simulink model "drone_failure_v3"  (R2021a)
settings: Solver=ode15s  StartTime=0.0  StopTime=35  FixedStep=0.1  RelTol=1e-3  EnableMultiTasking=on
settings Model: EnablePacing=on  PacingRate=1.100000  Creator=glembrez  LastModifiedBy=gabin
settings SolverCC: ZeroCrossAlgorithm=Adaptive  AlgebraicLoopSolver=TrustRegion  AutoInsertRateTranBlk=on
settings DataIOCC: LimitDataPoints=on
settings OptimizationCC: LifeSpan=inf
settings DebuggingCC: AllowSymbolicDim=off  SFUnexpectedBacktrackingDiag=warning  SFNoUnconditionalDefaultTransitionDiag=warning  SFExecutionAtInitializationDiag=none  ArithmeticOperatorsInVariantConditions=warning
settings SFSimCC: SimUseLocalCustomCode=off  CustomCodeUndefinedFunction=UseInterfaceOnly
settings RTWCC: RTWUseLocalCustomCode=off
settings CodeAppCC: StateflowObjectComments=on
settings GRTTargetCC: TargetLangStandard=C89/C90 (ANSI)
settings ConfigComp: CovMetricSettings=dw  CovSaveCumulativeToWorkspaceVar=on  CovSaveSingleToWorkspaceVar=on  CovExternalEMLEnable=off  CovSFcnEnable=off

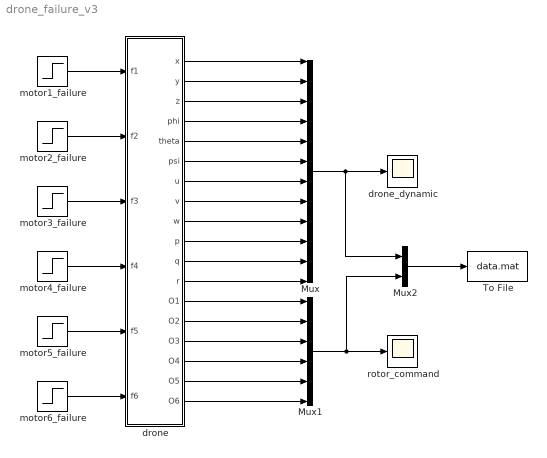
== system drone_failure_v3 ==
  Mux : Mux  Inputs=12
  Mux1 : Mux  Inputs=6
  Mux2 : Mux  Inputs=2
  To File : ToFile  Filename=data.mat  MatrixName=X  SaveFormat=Timeseries
  drone : Stateflow chart  TreatAsAtomicUnit=on
  drone_dynamic : Scope
  motor1_failure : Step  Time=10  SampleTime=0
  motor2_failure : Step  Time=35  SampleTime=0
  motor3_failure : Step  Time=35  SampleTime=0
  motor4_failure : Step  Time=35  SampleTime=0
  motor5_failure : Step  Time=35  SampleTime=0
  motor6_failure : Step  Time=35  SampleTime=0
  rotor_command : Scope
  wires:
  drone/1(x) -> Mux/1
  Mux/1 -> Mux2/1, drone_dynamic/1
  drone/2(y) -> Mux/2
  drone/3(z) -> Mux/3
  drone/4(phi) -> Mux/4
  drone/5(theta) -> Mux/5
  drone/6(psi) -> Mux/6
  drone/7(u) -> Mux/7
  drone/8(v) -> Mux/8
  drone/9(w) -> Mux/9
  drone/10(p) -> Mux/10
  drone/11(q) -> Mux/11
  drone/12(r) -> Mux/12
  drone/13(O1) -> Mux1/1
  drone/14(O2) -> Mux1/2
  drone/15(O3) -> Mux1/3
  drone/16(O4) -> Mux1/4
  drone/17(O5) -> Mux1/5
  drone/18(O6) -> Mux1/6
  Mux1/1 -> Mux2/2, rotor_command/1
  Mux2/1 -> To File/1
  motor2_failure/1 -> drone/2(f2)
  motor3_failure/1 -> drone/3(f3)
  motor4_failure/1 -> drone/4(f4)
  motor5_failure/1 -> drone/5(f5)
  motor6_failure/1 -> drone/6(f6)
  motor1_failure/1 -> drone/1(f1)

== stateflow chart drone_failure_v3/drone ==
  settings: updateMethod=CONTINUOUS
  state Drone
    state Normal_flight [parallel]
      %drone dynamic
      during:
      x_dot = cos(theta)*cos(psi)*u + (cos(psi)*sin(phi)*sin(theta)-cos(psi)*cos(phi))*v + (sin(phi)*sin(psi)+cos(phi)*cos(psi)*sin(theta))*w ;
      y_dot = cos(theta)*sin(psi)*u + (cos(theta)*cos(psi)+sin(phi)*sin(theta)*sin(psi))*v + (cos(phi)*sin(theta)*sin(psi)-sin(phi)*cos(psi))*w ;
      z_dot = -sin(theta)*u + cos(theta)*sin(phi)*v + cos(theta)*cos(phi)*w ;
      phi_dot = p+sin(phi)*tan(theta)*q+cos(phi)*tan(theta)*r ;
      theta_dot = cos(phi)*q - sin(phi)*r ;
      psi_dot = q*sin(phi)/cos(theta) + r*cos(phi)/cos(theta) ;
      u_dot = v*r-q*w-g*sin(theta)-u*(Kt+Kd*sqrt(u^2+v^2+w^2))/m ;
      v_dot = p*w-r*u+g*sin(phi)*cos(theta)-v*(Kt+Kd*sqrt(u^2+v^2+w^2))/m ;
      w_dot =q*u-p*v+g*cos(phi)*cos(theta)-w*Kd*sqrt(u^2+v^2+w^2)/m-(b*(O1^4+O2^4+O3^4+O4^4+O5^4+O6^4))/m;
      p_dot = q*r*(Iyy-Izz)/Ixx +((b*l/2 * (2*O2^4-2*O5^4+O1^4+O3^4-O4^4-O6^4))...
      -Jr*q*(-O1^2+O2^2-O3^2+O4^2-O5^2+O6^2))/Ixx;
      q_dot = p*r*(Izz-Ixx)/Iyy+((sqrt(3)*b*l/2 * (O1^4+O6^4-O3^4-O4^4))...
      +Jr*p*(-O1^2+O2^2-O3^2+O4^2-O5^2+O6^2))/Iyy ;
      r_dot = p*q*(Ixx-Iyy)/Izz+ (d*(O1^4-O2^4+O3^4-O4^4+O5^4-O6^4)...
      -Jr*2*(-O1*(O1c - O1)/0.01+O2*(O2c - O2)/0.01-O3*(O3c - O3)/0.01...
      +O4*(O4c - O4)/0.01-O5*(O5c - O5)/0.01+O6*(O6c - O6)/0.01))/Izz ;
      settings: executionOrder=1
    state Failure_detection [parallel]
      settings: executionOrder=2
      state fail4and2
        during:
        O1_dot = (O1c - O1)/tau+Kz*z-Kphi*phi+Ktheta*theta ;
        O2_dot = (O2c - O2)/tau ;
        O3_dot = (O3c - O3)/tau+Kz*z-Kphi*phi-Ktheta*theta ;
        O4_dot = (O4c - O4)/tau ;
        O5_dot = (O5c - O5)/tau +Kz*z+Kphi*phi ;;
        O6_dot = (O6c - O6)/tau+Kz*z+Kphi*phi+Ktheta*theta ;
      state fail1and5
        during:
        O1_dot = (O1c - O1)/tau ;
        O2_dot = (O2c - O2)/tau+Kz*z-Kphi*phi ;
        O3_dot = (O3c - O3)/tau+Kz*z-Kphi*phi-Ktheta*theta ;
        O4_dot = (O4c - O4)/tau+Kz*z-Kphi*phi-Ktheta*theta ;
        O5_dot = (O5c - O5)/tau ;
        O6_dot = (O6c - O6)/tau+Kz*z+Kphi*phi+Ktheta*theta ;
      state fail4
        during:
        O1_dot = (O1c - O1)/tau ;
        O2_dot = (O2c - O2)/tau+Kz*z-Kphi*phi ;
        O3_dot = (O3c - O3)/tau+Kz*z-Kphi*phi-Ktheta*theta ;
        O4_dot = (O4c - O4)/tau ;
        O5_dot = (O5c - O5)/tau+Kz*z+Kphi*phi ;
        O6_dot = (O6c - O6)/tau+Kz*z+Kphi*phi+Ktheta*theta ;
      state fail1
        during:
        O1_dot = (O1c - O1)/tau ;
        O2_dot = (O2c - O2)/tau+Kz*z-Kphi*phi ;
        O3_dot = (O3c - O3)/tau+Kz*z-Kphi*phi-Ktheta*theta ;
        O4_dot = (O4c - O4)/tau ;
        O5_dot = (O5c - O5)/tau+Kz*z+Kphi*phi ;
        O6_dot = (O6c - O6)/tau+Kz*z+Kphi*phi+Ktheta*theta ;
      state fail4and6
        during:
        O1_dot = (O1c - O1)/tau+Kz*z-Kphi*phi+Ktheta*theta ;
        O2_dot = (O2c - O2)/tau ;
        O3_dot = (O3c - O3)/tau+Kz*z-Kphi*phi-Ktheta*theta ;
        O4_dot = (O4c - O4)/tau ;
        O5_dot = (O5c - O5)/tau +Kz*z+Kphi*phi ;;
        O6_dot = (O6c - O6)/tau+Kz*z+Kphi*phi+Ktheta*theta ;
      state fail1and3
        during:
        O1_dot = (O1c - O1)/tau ;
        O2_dot = (O2c - O2)/tau+Kz*z-Kphi*phi ;
        O3_dot = (O3c - O3)/tau  ;
        O4_dot = (O4c - O4)/tau+Kz*z-Kphi*phi-Ktheta*theta ;
        O5_dot = (O5c - O5)/tau+Kz*z+Kphi*phi ;
        O6_dot = (O6c - O6)/tau+Kz*z+Kphi*phi+Ktheta*theta ;
      state fail2and4
        during:
        O1_dot = (O1c - O1)/tau+Kz*z-Kphi*phi+Ktheta*theta ;
        O2_dot = (O2c - O2)/tau ;
        O3_dot = (O3c - O3)/tau+Kz*z-Kphi*phi-Ktheta*theta ;
        O4_dot = (O4c - O4)/tau ;
        O5_dot = (O5c - O5)/tau +Kz*z+Kphi*phi ;;
        O6_dot = (O6c - O6)/tau+Kz*z+Kphi*phi+Ktheta*theta ;
      state fail5and1
        during:
        O1_dot = (O1c - O1)/tau ;
        O2_dot = (O2c - O2)/tau+Kz*z-Kphi*phi ;
        O3_dot = (O3c - O3)/tau+Kz*z-Kphi*phi-Ktheta*theta ;
        O4_dot = (O4c - O4)/tau+Kz*z-Kphi*phi-Ktheta*theta ;
        O5_dot = (O5c - O5)/tau ;
        O6_dot = (O6c - O6)/tau+Kz*z+Kphi*phi+Ktheta*theta ;
      state P_correction
        during:
        O1_dot = (O1c - O1)/tau+Kz*z-Kphi*phi+Ktheta*theta ;
        O2_dot = (O2c - O2)/tau+Kz*z-Kphi*phi ;
        O3_dot = (O3c - O3)/tau+Kz*z-Kphi*phi-Ktheta*theta ;
        O4_dot = (O4c - O4)/tau+Kz*z+Kphi*phi-Ktheta*theta ;
        O5_dot = (O5c - O5)/tau+Kz*z+Kphi*phi ;
        O6_dot = (O6c - O6)/tau+Kz*z+Kphi*phi+Ktheta*theta;
      state fail5
        during:
        O1_dot = (O1c - O1)/tau+Kz*z-Kphi*phi+Ktheta*theta ;
        O2_dot = (O2c - O2)/tau ;
        O3_dot = (O3c - O3)/tau+Kz*z-Kphi*phi-Ktheta*theta ;
        O4_dot = (O4c - O4)/tau+Kz*z+Kphi*phi-Ktheta*theta ;
        O5_dot = (O5c - O5)/tau ;
        O6_dot = (O6c - O6)/tau+Kz*z+Kphi*phi+Ktheta*theta ;
      state uncontrolable1
        during:
        O1_dot = (O1c - O1)/tau ;
        O2_dot = (O2c - O2)/tau ;
        O3_dot = (O3c - O3)/tau ;
        O4_dot = (O4c - O4)/tau ;
        O5_dot = (O5c - O5)/tau ;
        O6_dot = (O6c - O6)/tau;
      state fail2
        during:
        O1_dot = (O1c - O1)/tau+Kz*z-Kphi*phi+Ktheta*theta ;
        O2_dot = (O2c - O2)/tau ;
        O3_dot = (O3c - O3)/tau+Kz*z-Kphi*phi-Ktheta*theta ;
        O4_dot = (O4c - O4)/tau+Kz*z+Kphi*phi-Ktheta*theta ;
        O5_dot = (O5c - O5)/tau ;
        O6_dot = (O6c - O6)/tau+Kz*z+Kphi*phi+Ktheta*theta ;
      state uncontrolable
        during:
        O1_dot = (O1c - O1)/tau ;
        O2_dot = (O2c - O2)/tau ;
        O3_dot = (O3c - O3)/tau ;
        O4_dot = (O4c - O4)/tau ;
        O5_dot = (O5c - O5)/tau ;
        O6_dot = (O6c - O6)/tau;
      state fail5and3
        during:
        O1_dot = (O1c - O1)/tau+Kz*z-Kphi*phi+Ktheta*theta ;
        O2_dot = (O2c - O2)/tau+Kz*z-Kphi*phi ;
        O3_dot = (O3c - O3)/tau ;
        O4_dot = (O4c - O4)/tau+Kz*z+Kphi*phi-Ktheta*theta ;
        O5_dot = (O5c - O5)/tau ;
        O6_dot = (O6c - O6)/tau+Kz*z+Kphi*phi+Ktheta*theta ;
      state fail2and6
        during:
        O1_dot = (O1c - O1)/tau+Kz*z-Kphi*phi+Ktheta*theta ;
        O2_dot = (O2c - O2)/tau ;
        O3_dot = (O3c - O3)/tau+Kz*z-Kphi*phi-Ktheta*theta ;
        O4_dot = (O4c - O4)/tau+Kz*z+Kphi*phi-Ktheta*theta ;
        O5_dot = (O5c - O5)/tau +Kz*z+Kphi*phi ;
        O6_dot = (O6c - O6)/tau ;
      state fail3and1
        during:
        O1_dot = (O1c - O1)/tau ;
        O2_dot = (O2c - O2)/tau+Kz*z-Kphi*phi ;
        O3_dot = (O3c - O3)/tau  ;
        O4_dot = (O4c - O4)/tau+Kz*z-Kphi*phi-Ktheta*theta ;
        O5_dot = (O5c - O5)/tau+Kz*z+Kphi*phi ;
        O6_dot = (O6c - O6)/tau+Kz*z+Kphi*phi+Ktheta*theta ;
      state fail6and2
        during:
        O1_dot = (O1c - O1)/tau+Kz*z-Kphi*phi+Ktheta*theta ;
        O2_dot = (O2c - O2)/tau ;
        O3_dot = (O3c - O3)/tau+Kz*z-Kphi*phi-Ktheta*theta ;
        O4_dot = (O4c - O4)/tau+Kz*z+Kphi*phi-Ktheta*theta ;
        O5_dot = (O5c - O5)/tau +Kz*z+Kphi*phi ;
        O6_dot = (O6c - O6)/tau ;
      state fail6
        during:
        O1_dot = (O1c - O1)/tau+Kz*z-Kphi*phi+Ktheta*theta ;
        O2_dot = (O2c - O2)/tau+Kz*z-Kphi*phi ;
        O3_dot = (O3c - O3)/tau ;
        O4_dot = (O4c - O4)/tau+Kz*z+Kphi*phi-Ktheta*theta ;
        O5_dot = (O5c - O5)/tau+Kz*z+Kphi*phi ;
        O6_dot = (O6c - O6)/tau ;
      state fail3
        during:
        O1_dot = (O1c - O1)/tau+Kz*z-Kphi*phi+Ktheta*theta ;
        O2_dot = (O2c - O2)/tau+Kz*z-Kphi*phi ;
        O3_dot = (O3c - O3)/tau ;
        O4_dot = (O4c - O4)/tau+Kz*z+Kphi*phi-Ktheta*theta ;
        O5_dot = (O5c - O5)/tau+Kz*z+Kphi*phi ;
        O6_dot = (O6c - O6)/tau ;
      state fail3and5
        during:
        O1_dot = (O1c - O1)/tau+Kz*z-Kphi*phi+Ktheta*theta ;
        O2_dot = (O2c - O2)/tau+Kz*z-Kphi*phi ;
        O3_dot = (O3c - O3)/tau ;
        O4_dot = (O4c - O4)/tau+Kz*z+Kphi*phi-Ktheta*theta ;
        O5_dot = (O5c - O5)/tau ;
        O6_dot = (O6c - O6)/tau+Kz*z+Kphi*phi+Ktheta*theta ;
      state fail6and4
        during:
        O1_dot = (O1c - O1)/tau+Kz*z-Kphi*phi+Ktheta*theta ;
        O2_dot = (O2c - O2)/tau ;
        O3_dot = (O3c - O3)/tau+Kz*z-Kphi*phi-Ktheta*theta ;
        O4_dot = (O4c - O4)/tau ;
        O5_dot = (O5c - O5)/tau +Kz*z+Kphi*phi ;
        O6_dot = (O6c - O6)/tau+Kz*z+Kphi*phi+Ktheta*theta ;
      fail4and2 -> uncontrolable1 : [f1>eps|...
          | f6>eps|...
          | f3>eps|...
          | f5>eps]
          | {O1c= 0;
          | O2c = 0;
          | O3c = 0;
          | O4c = 0;
          | O5c = 0;
          | O6c = 0}
      fail1and5 -> uncontrolable : [f3>eps|...
          | f4>eps|...
          | f2>eps|...
          | f6>eps]
          | {O1c= 0;
          | O2c = 0;
          | O3c = 0;
          | O4c = 0;
          | O5c = 0;
          | O6c = 0}
      fail4 -> fail4and2 [order 1] : [f2>eps]{O1c=(m*g/(5*b))^(1/4);
          | O2c = 0;
          | O3c = (2^(1/4))*(m*g/(5*b))^(1/4);
          | O4c =  0;
          | O5c = (m*g/(5*b))^(1/4);
          | O6c = (m*g/(5*b))^(1/4)}
      fail1 -> fail1and5 [order 1] : [f5>eps]{O1c=0;
          | O2c = (m*g/(5*b))^(1/4);
          | O3c = (m*g/(5*b))^(1/4);
          | O4c =  (m*g/(5*b))^(1/4);
          | O5c = 0;
          | O6c = (2^(1/4))*(m*g/(5*b))^(1/4)}
      fail1 -> fail1 [order 4] : [f4>eps]
      fail4 -> uncontrolable1 [order 3] : [f3>eps|...
          | f5>eps]
          | {O1c= 0;
          | O2c = 0;
          | O3c = 0;
          | O4c = 0;
          | O5c = 0;
          | O6c = 0}
      P_correction -> fail1 [order 1] : [f1>eps]{O1c=0;
          | O2c = (m*g/(4*b))^(1/4);
          | O3c = (m*g/(4*b))^(1/4);
          | O4c = 0;
          | O5c = (m*g/(4*b))^(1/4);
          | O6c = (m*g/(4*b))^(1/4)}
      P_correction -> fail4 [order 4] : [f4>eps]{O1c=0;
          | O2c = (m*g/(4*b))^(1/4);
          | O3c = (m*g/(4*b))^(1/4);
          | O4c = 0;
          | O5c = (m*g/(4*b))^(1/4);
          | O6c = (m*g/(4*b))^(1/4)}
      fail1 -> uncontrolable [order 3] : [f6>eps|...
          | f2>eps]
          | {O1c= 0;
          | O2c = 0;
          | O3c = 0;
          | O4c = 0;
          | O5c = 0;
          | O6c = 0}
      fail4 -> fail4and6 [order 2] : [f6>eps]{O1c=(m*g/(5*b))^(1/4);
          | O2c = 0;
          | O3c = (m*g/(5*b))^(1/4);
          | O4c =  (m*g/(5*b))^(1/4);
          | O5c = (2^(1/4))*(m*g/(5*b))^(1/4);
          | O6c = 0}
      fail4 -> fail4 [order 4] : [f1>eps]
      fail1 -> fail1and3 [order 2] : [f3>eps]{O1c=0;
          | O2c = (2^(1/4))*(m*g/(5*b))^(1/4);
          | O3c = 0;
          | O4c =  (m*g/(5*b))^(1/4);
          | O5c = (m*g/(5*b))^(1/4);
          | O6c = (m*g/(5*b))^(1/4)}
      fail4and6 -> uncontrolable1 : [f1>eps|...
          | f2>eps|...
          | f3>eps|...
          | f5>eps]
          | {O1c= 0;
          | O2c = 0;
          | O3c = 0;
          | O4c = 0;
          | O5c = 0;
          | O6c = 0}
      fail1and3 -> uncontrolable : [f4>eps|...
          | f5>eps|...
          | f2>eps|...
          | f6>eps]
          | {O1c= 0;
          | O2c = 0;
          | O3c = 0;
          | O4c = 0;
          | O5c = 0;
          | O6c = 0}
      fail5 -> fail5and1 [order 1] : [f1>eps]{O1c=0;
          | O2c = (m*g/(5*b))^(1/4);
          | O3c = (m*g/(5*b))^(1/4);
          | O4c =  (m*g/(5*b))^(1/4);
          | O5c = 0;
          | O6c = (2^(1/4))*(m*g/(5*b))^(1/4)}
      fail2 -> fail2and4 [order 1] : [f4>eps]{O1c=(m*g/(5*b))^(1/4);
          | O2c = 0;
          | O3c = (2^(1/4))*(m*g/(5*b))^(1/4);
          | O4c =  0;
          | O5c = (m*g/(5*b))^(1/4);
          | O6c = (m*g/(5*b))^(1/4)}
      fail2 -> fail2 [order 4] : [f5>eps]
      fail5and1 -> uncontrolable1 : [f2>eps|...
          | f3>eps|...
          | f4>eps|...
          | f6>eps]
          | {O1c= 0;
          | O2c = 0;
          | O3c = 0;
          | O4c = 0;
          | O5c = 0;
          | O6c = 0}
      fail2and4 -> uncontrolable : [f5>eps|...
          | f6>eps|...
          | f1>eps|...
          | f3>eps]
          | {O1c= 0;
          | O2c = 0;
          | O3c = 0;
          | O4c = 0;
          | O5c = 0;
          | O6c = 0}
      (default) -> P_correction
      fail5 -> uncontrolable1 [order 3] : [f6>eps|...
          | f4>eps]
          | {O1c= 0;
          | O2c = 0;
          | O3c = 0;
          | O4c = 0;
          | O5c = 0;
          | O6c = 0}
      P_correction -> fail5 [order 5] : [f5>eps]{O1c=(m*g/(4*b))^(1/4);
          | O2c = 0;
          | O3c =  (m*g/(4*b))^(1/4);
          | O4c = (m*g/(4*b))^(1/4);
          | O5c = 0;
          | O6c = (m*g/(4*b))^(1/4)}
      fail5and3 -> uncontrolable1 : [f1>eps|...
          | f2>eps|...
          | f4>eps|...
          | f6>eps]
          | {O1c= 0;
          | O2c = 0;
          | O3c = 0;
          | O4c = 0;
          | O5c = 0;
          | O6c = 0}
      fail2 -> uncontrolable [order 3] : [f3>eps|...
          | f1>eps]
          | {O1c= 0;
          | O2c = 0;
          | O3c = 0;
          | O4c = 0;
          | O5c = 0;
          | O6c = 0}
      fail2and6 -> uncontrolable : [f4>eps|...
          | f5>eps|...
          | f1>eps|...
          | f3>eps]
          | {O1c= 0;
          | O2c = 0;
          | O3c = 0;
          | O4c = 0;
          | O5c = 0;
          | O6c = 0}
      P_correction -> fail2 [order 2] : [f2>eps]{O1c=(m*g/(4*b))^(1/4);
          | O2c = 0;
          | O3c =  (m*g/(4*b))^(1/4);
          | O4c = (m*g/(4*b))^(1/4);
          | O5c = 0;
          | O6c = (m*g/(4*b))^(1/4)}
      fail6 -> uncontrolable1 [order 3] : [f1>eps|...
          | f5>eps]
          | {O1c= 0;
          | O2c = 0;
          | O3c = 0;
          | O4c = 0;
          | O5c = 0;
          | O6c = 0}
      fail6and2 -> uncontrolable1 : [f1>eps|...
          | f3>eps|...
          | f4>eps|...
          | f5>eps]
          | {O1c= 0;
          | O2c = 0;
          | O3c = 0;
          | O4c = 0;
          | O5c = 0;
          | O6c = 0}
      fail6and4 -> uncontrolable1 : [f1>eps|...
          | f2>eps|...
          | f3>eps|...
          | f5>eps]
          | {O1c= 0;
          | O2c = 0;
          | O3c = 0;
          | O4c = 0;
          | O5c = 0;
          | O6c = 0}
      fail5 -> fail5and3 [order 2] : [f3>eps]{O1c=(m*g/(5*b))^(1/4);
          | O2c = (m*g/(5*b))^(1/4);
          | O3c = 0;
          | O4c = (2^(1/4))*(m*g/(5*b))^(1/4);
          | O5c = 0;
          | O6c = (m*g/(5*b))^(1/4)}
      fail5 -> fail5 [order 4] : [f2>eps]
      P_correction -> fail6 [order 6] : [f6>eps]{O1c=(m*g/(4*b))^(1/4);
          | O2c = (m*g/(4*b))^(1/4);
          | O3c = 0;
          | O4c = (m*g/(4*b))^(1/4);
          | O5c = (m*g/(4*b))^(1/4);
          | O6c = 0}
      P_correction -> fail3 [order 3] : [f3>eps]{O1c=(m*g/(4*b))^(1/4);
          | O2c = (m*g/(4*b))^(1/4);
          | O3c = 0;
          | O4c = (m*g/(4*b))^(1/4);
          | O5c = (m*g/(4*b))^(1/4);
          | O6c = 0}
      fail3 -> uncontrolable [order 4] : [f2>eps|...
          | f4>eps]
          | {O1c= 0;
          | O2c = 0;
          | O3c = 0;
          | O4c = 0;
          | O5c = 0;
          | O6c = 0}
      fail3and1 -> uncontrolable : [f5>eps|...
          | f6>eps|...
          | f2>eps|...
          | f4>eps]
          | {O1c= 0;
          | O2c = 0;
          | O3c = 0;
          | O4c = 0;
          | O5c = 0;
          | O6c = 0}
      fail3and5 -> uncontrolable : [f1>eps|...
          | f6>eps|...
          | f2>eps|...
          | f4>eps]
          | {O1c= 0;
          | O2c = 0;
          | O3c = 0;
          | O4c = 0;
          | O5c = 0;
          | O6c = 0}
      fail2 -> fail2and6 [order 2] : [f6>eps]{O1c=(2^(1/4))*(m*g/(5*b))^(1/4);
          | O2c = 0;
          | O3c = (m*g/(5*b))^(1/4);
          | O4c = (m*g/(5*b))^(1/4);
          | O5c = (m*g/(5*b))^(1/4);
          | O6c = 0;}
      fail6 -> fail6and2 [order 1] : [f2>eps]{O1c=(2^(1/4))*(m*g/(5*b))^(1/4);
          | O2c = 0;
          | O3c = (m*g/(5*b))^(1/4);
          | O4c = (m*g/(5*b))^(1/4);
          | O5c = (m*g/(5*b))^(1/4);
          | O6c = 0;}
      fail3 -> fail3and1 [order 1] : [f1>eps]{O1c=0;
          | O2c = (2^(1/4))*(m*g/(5*b))^(1/4);
          | O3c = 0;
          | O4c =  (m*g/(5*b))^(1/4);
          | O5c = (m*g/(5*b))^(1/4);
          | O6c = (m*g/(5*b))^(1/4)}
      fail3 -> fail3 [order 3] : [f6>eps]
      fail6 -> fail6and4 [order 2] : [f4>eps]{O1c=(m*g/(5*b))^(1/4);
          | O2c = 0;
          | O3c = (m*g/(5*b))^(1/4);
          | O4c =  (m*g/(5*b))^(1/4);
          | O5c = (2^(1/4))*(m*g/(5*b))^(1/4);
          | O6c = 0}
      fail6 -> fail6 [order 4] : [f3>eps]
      fail3 -> fail3and5 [order 2] : [f5>eps]{O1c=(m*g/(5*b))^(1/4);
          | O2c = (m*g/(5*b))^(1/4);
          | O3c = 0;
          | O4c =  (2^(1/4))*(m*g/(5*b))^(1/4);
          | O5c = 0;
          | O6c = (m*g/(5*b))^(1/4)}
  data: Ixx local =5.126e-3; Iyy local =5.126e-3; Izz local =1.3e-2; l local =0.5; d local =1.140e-7; g local =9.81; m local =2.4; Kd local =7.5e-3; Kt local =3.13e-5; b local =2.9e-5; x output =0; y output =0; z output =0; phi output =0; theta output =0; psi output =0; u output =0; v output =0; w output =0; p output =0; q output =0; r output =0; Jr local =4.2e-6; M_phi local =0; M_theta local =0; M_psi local =0; O_R local =0; O_R_d local =0; O1c local =19.05; O2c local =19.05; O3c local =19.05; O4c local =19.05; O5c local =19.05; O6c local =19.05; O1 output =19.05; O2 output =19.05; O3 output =19.05; O4 output =19.05; O5 output =19.05; O6 output =19.05; Tt local =23.544; Kz local =1; eps local =0.5; tau local =0.1; Kphi local =0.01; Ktheta local =-0.01; f1 input; f2 input; f3 input; f4 input; f5 input; f6 input
  data x settings: updateMethod=SF_CONTINUOUS_TIME_DATA
  data y settings: updateMethod=SF_CONTINUOUS_TIME_DATA
  data z settings: updateMethod=SF_CONTINUOUS_TIME_DATA
  data phi settings: updateMethod=SF_CONTINUOUS_TIME_DATA
  data theta settings: updateMethod=SF_CONTINUOUS_TIME_DATA
  data psi settings: updateMethod=SF_CONTINUOUS_TIME_DATA
  data u settings: updateMethod=SF_CONTINUOUS_TIME_DATA
  data v settings: updateMethod=SF_CONTINUOUS_TIME_DATA
  data w settings: updateMethod=SF_CONTINUOUS_TIME_DATA
  data p settings: updateMethod=SF_CONTINUOUS_TIME_DATA
  data q settings: updateMethod=SF_CONTINUOUS_TIME_DATA
  data r settings: updateMethod=SF_CONTINUOUS_TIME_DATA
  data O1 settings: updateMethod=SF_CONTINUOUS_TIME_DATA
  data O2 settings: updateMethod=SF_CONTINUOUS_TIME_DATA
  data O3 settings: updateMethod=SF_CONTINUOUS_TIME_DATA
  data O4 settings: updateMethod=SF_CONTINUOUS_TIME_DATA
  data O5 settings: updateMethod=SF_CONTINUOUS_TIME_DATA
  data O6 settings: updateMethod=SF_CONTINUOUS_TIME_DATA
